simulink model "OPSKBasedCommunicationModel"  (R2023a)
settings: Solver=ode45  StartTime=0.0  StopTime=10.0  RelTol=1e-3
libraries: commsrccod2 x2, commdigbbndpm3 x2, commrandsrc3 x1
settings Model: Creator=paragmraw  LastModifiedBy=paragmraw

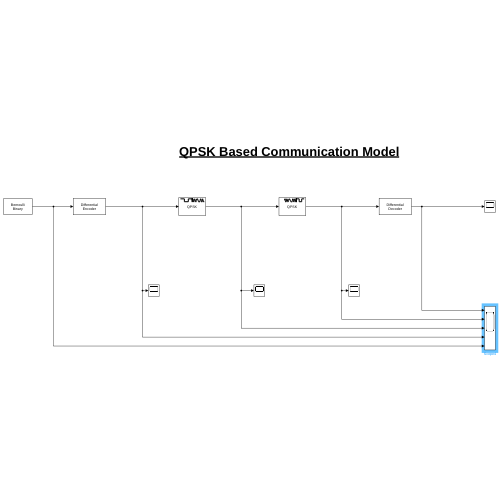
[thumbnail: Simulink's stored preview of the top-level diagram]
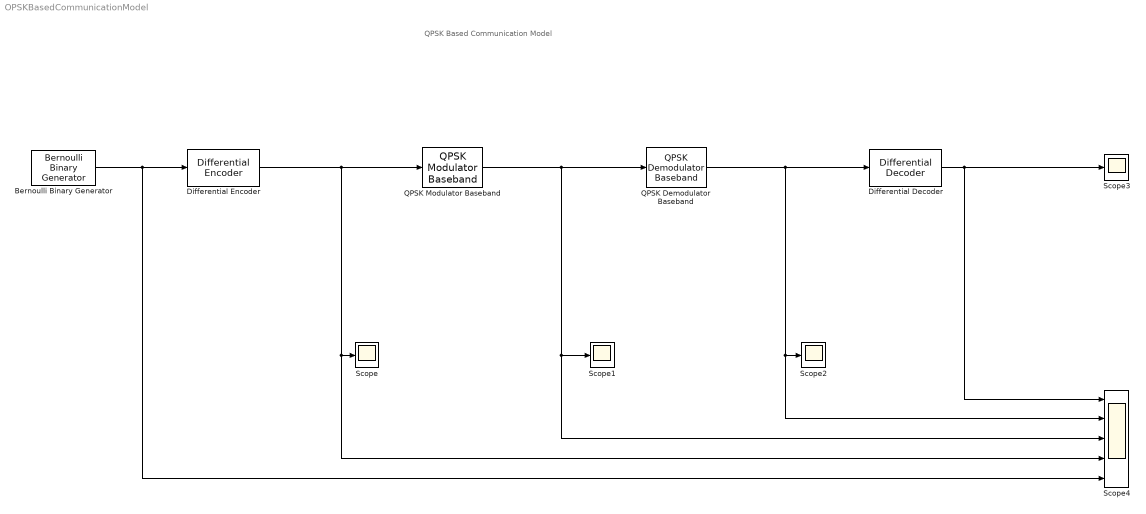
== system OPSKBasedCommunicationModel ==
  note: QPSK Based Communication Model
  Bernoulli Binary Generator : commrandsrc3/Bernoulli Binary Generator  ProbabilityOfZero=0.5  SeedSource=Parameter  Seed=0  SampleTime=1  SamplesPerFrame=1  OutputDataType=double  SimulateUsing=Interpreted execution
  Differential Decoder : commsrccod2/Differential Decoder  InitCond=0
  Differential Encoder : commsrccod2/Differential Encoder  InitCond=0
  QPSK Demodulator Baseband : commdigbbndpm3/QPSK Demodulator Baseband  OutType=Integer  DecType=Hard decision  VarSource=Dialog  Variance=1  Dec=Gray  Ph=pi/4  outDtype1=Inherit via internal rule  outDtype2=Inherit via internal rule  derotateFactorWordLen=16  derotateFactorDataTypeStr=Inherit: Same word length as input  derotateFactorLastDataTypeStr=Inherit: Same word length as input
  QPSK Modulator Baseband : commdigbbndpm3/QPSK Modulator Baseband  InType=Integer  Enc=Gray  Ph=pi/4  outDtype=double  outWordLen=16  outUDDataType=sfix(16)  outFracLenMode=Best precision  outFracLen=15  outDataTypeStr=double  outLastDataTypeStr=double
  Scope{,1..3} (4 alike) : Scope
  Scope4 : Scope  NumInputPorts=5
  wires:
  Bernoulli Binary Generator/1 -> Scope4/5, Differential Encoder/1
  Differential Encoder/1 -> QPSK Modulator Baseband/1, Scope4/4, Scope/1
  QPSK Modulator Baseband/1 -> Scope1/1, Scope4/3, QPSK Demodulator Baseband/1
  QPSK Demodulator Baseband/1 -> Scope4/2, Scope2/1, Differential Decoder/1
  Differential Decoder/1 -> Scope4/1, Scope3/1
